simulink model "CryoDetHcd"  (R2016b)
settings: Solver=ode45  StartTime=0.0  StopTime=1e-3  RelTol=1e-3
PreLoadFcn:
  | setup_hcd
values from neighbouring files (symbols this model uses):
  A = sqrt(0.5*erfc(x))    [setup_hcd.m]
  etaRomData = zeros(1,128)    [setup_hcd.m]
  Fadc = 614e6    (= 614000000)    [setup_hcd.m]
  freqRomData = zeros(1,128)    [setup_hcd.m]
  freqRomData1 = zeros(1,128)    [setup_hcd.m]
  freqRomData2 = zeros(1,128)    [setup_hcd.m]
  freqRomData3 = zeros(1,128)    [setup_hcd.m]
undefined symbols (not defined in the file or in its folder): AXI4, B, C, D, j, Lite
libraries: xbsIndex_r4 x2151, CryoDetLibCMB x28, hdlsllib x8, dspsigops x2, simulink x1
(part 8 of 17)

== system CryoDetHcd/DspCore/DSP/channel_processor/channel_processor_x4/128_channel_processor1/DDS Mixer taylor series corrected ==
  rst : Inport
  In : Inport  Port=2
  freqBus : Inport  Port=3
  index : Inport  Port=4
  Bus Creator1 : BusCreator  Inputs=4
  Bus Creator2 : BusCreator  Inputs=5
  Bus Selector1 : BusSelector  OutputSignals=valid,Q,I,amp,ch
  Bus Selector2 : BusSelector  OutputSignals=valid
  Bus Selector : BusSelector  OutputSignals=freqWord,ch
  DDS 8ch taylor series corrected : Subsystem  AncestorBlock=CryoDetLibCMB/DDS 8ch taylor series corrected
  IQ_scale : CryoDetLibCMB/IQ_scale
  mixer : Subsystem
  tones : Outport
  downconvert : Outport  Port=2
  phase : Outport  Port=3
  wires:
  rst/1 -> DDS 8ch taylor series corrected/2(rst)
  Bus Selector/1 -> DDS 8ch taylor series corrected/3(freqWord)  "<freqWord>"
  Bus Selector1/5 -> IQ_scale/5  "<ch>"
  Bus Selector1/4 -> IQ_scale/4  "<amp>"
  DDS 8ch taylor series corrected/4(amp_o) -> Bus Creator2/4  "amp"
  DDS 8ch taylor series corrected/5(ch_o) -> Bus Creator2/5  "ch"
  In/1 -> Bus Selector2/1, mixer/2(In2)
  freqBus/1 -> Bus Selector/1
  Bus Selector2/1 -> DDS 8ch taylor series corrected/1(valid)  "<valid>"
  index/1 -> DDS 8ch taylor series corrected/4(index)
  IQ_scale/1 -> Bus Creator1/1  "valid"
  IQ_scale/2 -> Bus Creator1/2  "Q"
  IQ_scale/3 -> Bus Creator1/3  "I"
  IQ_scale/4 -> Bus Creator1/4  "ch"
  Bus Creator1/1 -> tones/1
  DDS 8ch taylor series corrected/3(I) -> Bus Creator2/3  "I"
  DDS 8ch taylor series corrected/1(valid_o) -> Bus Creator2/1  "valid"
  DDS 8ch taylor series corrected/2(Q) -> Bus Creator2/2  "Q"
  Bus Creator2/1 -> mixer/1(In1), Bus Selector1/1
  Bus Selector1/3 -> IQ_scale/3  "<I>"
  Bus Selector1/2 -> IQ_scale/2  "<Q>"
  Bus Selector1/1 -> IQ_scale/1  "<valid>"
  Bus Selector/2 -> DDS 8ch taylor series corrected/5(ch)  "<ch>"
  mixer/1(downmix) -> downconvert/1  "valid"
  mixer/2(phaseBus_o) -> phase/1
  DDS 8ch taylor series corrected/6(phaseBus) -> mixer/3(phaseBus)

== system CryoDetHcd/DspCore/DSP/channel_processor/channel_processor_x4/128_channel_processor1/IQ_status_sel ==
  sel : Inport
  Q : Inport  Port=2
  I : Inport  Port=3
  ch : Inport  Port=4
  BitBasher : xbsIndex_r4/BitBasher  bitexpr=out = {I,Q}  display_expr=off  sr_1=out  arith_type1=Unsigned  bin_pt1=0  sr_2=2  arith_type2=Unsigned  bin_pt2=0  sr_3=3  arith_type3=Unsigned  bin_pt3=0  sr_4=4  arith_type4=Unsigned  bin_pt4=0  dbl_ovrd=off  block_type=bitbasher
  Convert : xbsIndex_r4/Convert  gui_display_data_type=Fixed-point  arith_type="Signed  (2's comp)"  n_bits=16  bin_pt=15  float_type=Single  exp_bits=8  fraction_bits=24  quantization=Truncate  overflow=Wrap  en=off  latency=1  pipeline=off  dbl_ovrd=off  block_type=convert
  Convert1 : xbsIndex_r4/Convert  gui_display_data_type=Fixed-point  arith_type="Signed  (2's comp)"  n_bits=16  bin_pt=15  float_type=Single  exp_bits=8  fraction_bits=24  quantization=Truncate  overflow=Wrap  en=off  latency=1  pipeline=off  dbl_ovrd=off  block_type=convert
  Register1 : xbsIndex_r4/Register  init=0  rst=off  en=on  dbl_ovrd=off  block_type=register
  Relational : xbsIndex_r4/Relational  mode=a=b  op_type=Bool  en=off  latency=1  dbl_ovrd=off  block_type=relational
  IQ_status_r : Outport
  wires:
  sel/1 -> Relational/1
  Convert/1 -> BitBasher/1
  ch/1 -> Relational/2
  Q/1 -> Convert/1
  I/1 -> Convert1/1
  BitBasher/1 -> Register1/1
  Register1/1 -> IQ_status_r/1
  Convert1/1 -> BitBasher/2
  Relational/1 -> Register1/2

== system CryoDetHcd/DspCore/DSP/channel_processor/channel_processor_x4/128_channel_processor1/Variant Subsystem ==
  note: 1) Add Subsystem or Model blocks as valid variant choices.
      | 2) You cannot connect blocks at this level. At simulation, connectivity is automatically
      | determined, based on the active variant and port name matching.
  valid : Inport
  feedbackPolarity : Inport  Port=2
  feedbackGain : Inport  Port=3
  feedbackLimitHi : Inport  Port=4
  feedbackLimitLo : Inport  Port=5
  freqError : Inport  Port=6
  freqWord : Inport  Port=7
  ch : Inport  Port=8
  reset : Inport  Port=9
  LMS : Subsystem  AncestorBlock=CryoDetLibCMB/Loop Filter1  VariantControl=Variant
  Loop Filter1 : CryoDetLibCMB/Loop Filter1  VariantControl=Variant1
      link override Delay: rst=off  infoeditControl=Selection of Reset will increase slice count due to use of real FFs and instead of SRLs  en=off  latency=1  reg_retiming=off  dbl_ovrd=off
      link override Delay: infoedit=Hardware notes: A delay line is a chain, each link of which is an SRL16 followed by a flip-flop.
  valid_o : Outport
  freqWordOut : Outport  Port=2
  ch_o : Outport  Port=3

== system CryoDetHcd/DspCore/DSP/channel_processor/channel_processor_x4/128_channel_processor2/DDS Mixer taylor series corrected ==
  rst : Inport
  In : Inport  Port=2
  freqBus : Inport  Port=3
  index : Inport  Port=4
  Bus Creator1 : BusCreator  Inputs=4
  Bus Creator2 : BusCreator  Inputs=5
  Bus Selector1 : BusSelector  OutputSignals=valid,Q,I,amp,ch
  Bus Selector2 : BusSelector  OutputSignals=valid
  Bus Selector : BusSelector  OutputSignals=freqWord,ch
  DDS 8ch taylor series corrected : Subsystem  AncestorBlock=CryoDetLibCMB/DDS 8ch taylor series corrected
  IQ_scale : CryoDetLibCMB/IQ_scale
  mixer : Subsystem
  tones : Outport
  downconvert : Outport  Port=2
  phase : Outport  Port=3
  wires:
  DDS 8ch taylor series corrected/6(phaseBus) -> mixer/3(phaseBus)
  mixer/2(phaseBus_o) -> phase/1
  mixer/1(downmix) -> downconvert/1  "valid"
  Bus Selector/2 -> DDS 8ch taylor series corrected/5(ch)  "<ch>"
  Bus Selector1/1 -> IQ_scale/1  "<valid>"
  Bus Selector1/2 -> IQ_scale/2  "<Q>"
  Bus Selector1/3 -> IQ_scale/3  "<I>"
  Bus Creator2/1 -> Bus Selector1/1, mixer/1(In1)
  DDS 8ch taylor series corrected/2(Q) -> Bus Creator2/2  "Q"
  DDS 8ch taylor series corrected/1(valid_o) -> Bus Creator2/1  "valid"
  DDS 8ch taylor series corrected/3(I) -> Bus Creator2/3  "I"
  Bus Creator1/1 -> tones/1
  IQ_scale/4 -> Bus Creator1/4  "ch"
  IQ_scale/3 -> Bus Creator1/3  "I"
  IQ_scale/2 -> Bus Creator1/2  "Q"
  IQ_scale/1 -> Bus Creator1/1  "valid"
  index/1 -> DDS 8ch taylor series corrected/4(index)
  Bus Selector2/1 -> DDS 8ch taylor series corrected/1(valid)  "<valid>"
  freqBus/1 -> Bus Selector/1
  In/1 -> mixer/2(In2), Bus Selector2/1
  DDS 8ch taylor series corrected/5(ch_o) -> Bus Creator2/5  "ch"
  DDS 8ch taylor series corrected/4(amp_o) -> Bus Creator2/4  "amp"
  Bus Selector1/4 -> IQ_scale/4  "<amp>"
  Bus Selector1/5 -> IQ_scale/5  "<ch>"
  Bus Selector/1 -> DDS 8ch taylor series corrected/3(freqWord)  "<freqWord>"
  rst/1 -> DDS 8ch taylor series corrected/2(rst)

== system CryoDetHcd/DspCore/DSP/channel_processor/channel_processor_x4/128_channel_processor2/IQ_status_sel ==
  sel : Inport
  Q : Inport  Port=2
  I : Inport  Port=3
  ch : Inport  Port=4
  BitBasher : xbsIndex_r4/BitBasher  bitexpr=out = {I,Q}  display_expr=off  sr_1=out  arith_type1=Unsigned  bin_pt1=0  sr_2=2  arith_type2=Unsigned  bin_pt2=0  sr_3=3  arith_type3=Unsigned  bin_pt3=0  sr_4=4  arith_type4=Unsigned  bin_pt4=0  dbl_ovrd=off  block_type=bitbasher
  Convert : xbsIndex_r4/Convert  gui_display_data_type=Fixed-point  arith_type="Signed  (2's comp)"  n_bits=16  bin_pt=15  float_type=Single  exp_bits=8  fraction_bits=24  quantization=Truncate  overflow=Wrap  en=off  latency=1  pipeline=off  dbl_ovrd=off  block_type=convert
  Convert1 : xbsIndex_r4/Convert  gui_display_data_type=Fixed-point  arith_type="Signed  (2's comp)"  n_bits=16  bin_pt=15  float_type=Single  exp_bits=8  fraction_bits=24  quantization=Truncate  overflow=Wrap  en=off  latency=1  pipeline=off  dbl_ovrd=off  block_type=convert
  Register1 : xbsIndex_r4/Register  init=0  rst=off  en=on  dbl_ovrd=off  block_type=register
  Relational : xbsIndex_r4/Relational  mode=a=b  op_type=Bool  en=off  latency=1  dbl_ovrd=off  block_type=relational
  IQ_status_r : Outport
  wires:
  Relational/1 -> Register1/2
  Convert1/1 -> BitBasher/2
  Register1/1 -> IQ_status_r/1
  BitBasher/1 -> Register1/1
  I/1 -> Convert1/1
  Q/1 -> Convert/1
  ch/1 -> Relational/2
  Convert/1 -> BitBasher/1
  sel/1 -> Relational/1

== system CryoDetHcd/DspCore/DSP/channel_processor/channel_processor_x4/128_channel_processor2/Variant Subsystem ==
  note: 1) Add Subsystem or Model blocks as valid variant choices.
      | 2) You cannot connect blocks at this level. At simulation, connectivity is automatically
      | determined, based on the active variant and port name matching.
  valid : Inport
  feedbackPolarity : Inport  Port=2
  feedbackGain : Inport  Port=3
  feedbackLimitHi : Inport  Port=4
  feedbackLimitLo : Inport  Port=5
  freqError : Inport  Port=6
  freqWord : Inport  Port=7
  ch : Inport  Port=8
  reset : Inport  Port=9
  LMS : Subsystem  AncestorBlock=CryoDetLibCMB/Loop Filter1  VariantControl=Variant
  Loop Filter1 : CryoDetLibCMB/Loop Filter1  VariantControl=Variant1
      link override Delay: rst=off  infoeditControl=Selection of Reset will increase slice count due to use of real FFs and instead of SRLs  en=off  latency=1  reg_retiming=off  dbl_ovrd=off
      link override Delay: infoedit=Hardware notes: A delay line is a chain, each link of which is an SRL16 followed by a flip-flop.
  valid_o : Outport
  freqWordOut : Outport  Port=2
  ch_o : Outport  Port=3

== system CryoDetHcd/DspCore/DSP/channel_processor/channel_processor_x4/128_channel_processor3/DDS Mixer taylor series corrected ==
  rst : Inport
  In : Inport  Port=2
  freqBus : Inport  Port=3
  index : Inport  Port=4
  Bus Creator1 : BusCreator  Inputs=4
  Bus Creator2 : BusCreator  Inputs=5
  Bus Selector1 : BusSelector  OutputSignals=valid,Q,I,amp,ch
  Bus Selector2 : BusSelector  OutputSignals=valid
  Bus Selector : BusSelector  OutputSignals=freqWord,ch
  DDS 8ch taylor series corrected : Subsystem  AncestorBlock=CryoDetLibCMB/DDS 8ch taylor series corrected
  IQ_scale : CryoDetLibCMB/IQ_scale
  mixer : Subsystem
  tones : Outport
  downconvert : Outport  Port=2
  phase : Outport  Port=3
  wires:
  rst/1 -> DDS 8ch taylor series corrected/2(rst)
  Bus Selector/1 -> DDS 8ch taylor series corrected/3(freqWord)  "<freqWord>"
  Bus Selector1/5 -> IQ_scale/5  "<ch>"
  Bus Selector1/4 -> IQ_scale/4  "<amp>"
  DDS 8ch taylor series corrected/4(amp_o) -> Bus Creator2/4  "amp"
  DDS 8ch taylor series corrected/5(ch_o) -> Bus Creator2/5  "ch"
  In/1 -> Bus Selector2/1, mixer/2(In2)
  freqBus/1 -> Bus Selector/1
  Bus Selector2/1 -> DDS 8ch taylor series corrected/1(valid)  "<valid>"
  index/1 -> DDS 8ch taylor series corrected/4(index)
  IQ_scale/1 -> Bus Creator1/1  "valid"
  IQ_scale/2 -> Bus Creator1/2  "Q"
  IQ_scale/3 -> Bus Creator1/3  "I"
  IQ_scale/4 -> Bus Creator1/4  "ch"
  Bus Creator1/1 -> tones/1
  DDS 8ch taylor series corrected/3(I) -> Bus Creator2/3  "I"
  DDS 8ch taylor series corrected/1(valid_o) -> Bus Creator2/1  "valid"
  DDS 8ch taylor series corrected/2(Q) -> Bus Creator2/2  "Q"
  Bus Creator2/1 -> mixer/1(In1), Bus Selector1/1
  Bus Selector1/3 -> IQ_scale/3  "<I>"
  Bus Selector1/2 -> IQ_scale/2  "<Q>"
  Bus Selector1/1 -> IQ_scale/1  "<valid>"
  Bus Selector/2 -> DDS 8ch taylor series corrected/5(ch)  "<ch>"
  mixer/1(downmix) -> downconvert/1  "valid"
  mixer/2(phaseBus_o) -> phase/1
  DDS 8ch taylor series corrected/6(phaseBus) -> mixer/3(phaseBus)

== system CryoDetHcd/DspCore/DSP/channel_processor/channel_processor_x4/128_channel_processor3/IQ_status_sel ==
  sel : Inport
  Q : Inport  Port=2
  I : Inport  Port=3
  ch : Inport  Port=4
  BitBasher : xbsIndex_r4/BitBasher  bitexpr=out = {I,Q}  display_expr=off  sr_1=out  arith_type1=Unsigned  bin_pt1=0  sr_2=2  arith_type2=Unsigned  bin_pt2=0  sr_3=3  arith_type3=Unsigned  bin_pt3=0  sr_4=4  arith_type4=Unsigned  bin_pt4=0  dbl_ovrd=off  block_type=bitbasher
  Convert : xbsIndex_r4/Convert  gui_display_data_type=Fixed-point  arith_type="Signed  (2's comp)"  n_bits=16  bin_pt=15  float_type=Single  exp_bits=8  fraction_bits=24  quantization=Truncate  overflow=Wrap  en=off  latency=1  pipeline=off  dbl_ovrd=off  block_type=convert
  Convert1 : xbsIndex_r4/Convert  gui_display_data_type=Fixed-point  arith_type="Signed  (2's comp)"  n_bits=16  bin_pt=15  float_type=Single  exp_bits=8  fraction_bits=24  quantization=Truncate  overflow=Wrap  en=off  latency=1  pipeline=off  dbl_ovrd=off  block_type=convert
  Register1 : xbsIndex_r4/Register  init=0  rst=off  en=on  dbl_ovrd=off  block_type=register
  Relational : xbsIndex_r4/Relational  mode=a=b  op_type=Bool  en=off  latency=1  dbl_ovrd=off  block_type=relational
  IQ_status_r : Outport
  wires:
  sel/1 -> Relational/1
  Convert/1 -> BitBasher/1
  ch/1 -> Relational/2
  Q/1 -> Convert/1
  I/1 -> Convert1/1
  BitBasher/1 -> Register1/1
  Register1/1 -> IQ_status_r/1
  Convert1/1 -> BitBasher/2
  Relational/1 -> Register1/2

== system CryoDetHcd/DspCore/DSP/channel_processor/channel_processor_x4/128_channel_processor3/Variant Subsystem ==
  note: 1) Add Subsystem or Model blocks as valid variant choices.
      | 2) You cannot connect blocks at this level. At simulation, connectivity is automatically
      | determined, based on the active variant and port name matching.
  valid : Inport
  feedbackPolarity : Inport  Port=2
  feedbackGain : Inport  Port=3
  feedbackLimitHi : Inport  Port=4
  feedbackLimitLo : Inport  Port=5
  freqError : Inport  Port=6
  freqWord : Inport  Port=7
  ch : Inport  Port=8
  reset : Inport  Port=9
  LMS : Subsystem  AncestorBlock=CryoDetLibCMB/Loop Filter1  VariantControl=Variant
  Loop Filter1 : CryoDetLibCMB/Loop Filter1  VariantControl=Variant1
      link override Delay: rst=off  infoeditControl=Selection of Reset will increase slice count due to use of real FFs and instead of SRLs  en=off  latency=1  reg_retiming=off  dbl_ovrd=off
      link override Delay: infoedit=Hardware notes: A delay line is a chain, each link of which is an SRL16 followed by a flip-flop.
  valid_o : Outport
  freqWordOut : Outport  Port=2
  ch_o : Outport  Port=3

== system CryoDetHcd/DspCore/DSP/channel_processor/channel_processor_x4/128_channel_processor4/DDS Mixer taylor series corrected ==
  rst : Inport
  In : Inport  Port=2
  freqBus : Inport  Port=3
  index : Inport  Port=4
  Bus Creator1 : BusCreator  Inputs=4
  Bus Creator2 : BusCreator  Inputs=5
  Bus Selector1 : BusSelector  OutputSignals=valid,Q,I,amp,ch
  Bus Selector2 : BusSelector  OutputSignals=valid
  Bus Selector : BusSelector  OutputSignals=freqWord,ch
  DDS 8ch taylor series corrected : Subsystem  AncestorBlock=CryoDetLibCMB/DDS 8ch taylor series corrected
  IQ_scale : CryoDetLibCMB/IQ_scale
  mixer : Subsystem
  tones : Outport
  downconvert : Outport  Port=2
  phase : Outport  Port=3
  wires:
  DDS 8ch taylor series corrected/6(phaseBus) -> mixer/3(phaseBus)
  mixer/2(phaseBus_o) -> phase/1
  mixer/1(downmix) -> downconvert/1  "valid"
  Bus Selector/2 -> DDS 8ch taylor series corrected/5(ch)  "<ch>"
  Bus Selector1/1 -> IQ_scale/1  "<valid>"
  Bus Selector1/2 -> IQ_scale/2  "<Q>"
  Bus Selector1/3 -> IQ_scale/3  "<I>"
  Bus Creator2/1 -> Bus Selector1/1, mixer/1(In1)
  DDS 8ch taylor series corrected/2(Q) -> Bus Creator2/2  "Q"
  DDS 8ch taylor series corrected/1(valid_o) -> Bus Creator2/1  "valid"
  DDS 8ch taylor series corrected/3(I) -> Bus Creator2/3  "I"
  Bus Creator1/1 -> tones/1
  IQ_scale/4 -> Bus Creator1/4  "ch"
  IQ_scale/3 -> Bus Creator1/3  "I"
  IQ_scale/2 -> Bus Creator1/2  "Q"
  IQ_scale/1 -> Bus Creator1/1  "valid"
  index/1 -> DDS 8ch taylor series corrected/4(index)
  Bus Selector2/1 -> DDS 8ch taylor series corrected/1(valid)  "<valid>"
  freqBus/1 -> Bus Selector/1
  In/1 -> mixer/2(In2), Bus Selector2/1
  DDS 8ch taylor series corrected/5(ch_o) -> Bus Creator2/5  "ch"
  DDS 8ch taylor series corrected/4(amp_o) -> Bus Creator2/4  "amp"
  Bus Selector1/4 -> IQ_scale/4  "<amp>"
  Bus Selector1/5 -> IQ_scale/5  "<ch>"
  Bus Selector/1 -> DDS 8ch taylor series corrected/3(freqWord)  "<freqWord>"
  rst/1 -> DDS 8ch taylor series corrected/2(rst)

== system CryoDetHcd/DspCore/DSP/channel_processor/channel_processor_x4/128_channel_processor4/IQ_status_sel ==
  sel : Inport
  Q : Inport  Port=2
  I : Inport  Port=3
  ch : Inport  Port=4
  BitBasher : xbsIndex_r4/BitBasher  bitexpr=out = {I,Q}  display_expr=off  sr_1=out  arith_type1=Unsigned  bin_pt1=0  sr_2=2  arith_type2=Unsigned  bin_pt2=0  sr_3=3  arith_type3=Unsigned  bin_pt3=0  sr_4=4  arith_type4=Unsigned  bin_pt4=0  dbl_ovrd=off  block_type=bitbasher
  Convert : xbsIndex_r4/Convert  gui_display_data_type=Fixed-point  arith_type="Signed  (2's comp)"  n_bits=16  bin_pt=15  float_type=Single  exp_bits=8  fraction_bits=24  quantization=Truncate  overflow=Wrap  en=off  latency=1  pipeline=off  dbl_ovrd=off  block_type=convert
  Convert1 : xbsIndex_r4/Convert  gui_display_data_type=Fixed-point  arith_type="Signed  (2's comp)"  n_bits=16  bin_pt=15  float_type=Single  exp_bits=8  fraction_bits=24  quantization=Truncate  overflow=Wrap  en=off  latency=1  pipeline=off  dbl_ovrd=off  block_type=convert
  Register1 : xbsIndex_r4/Register  init=0  rst=off  en=on  dbl_ovrd=off  block_type=register
  Relational : xbsIndex_r4/Relational  mode=a=b  op_type=Bool  en=off  latency=1  dbl_ovrd=off  block_type=relational
  IQ_status_r : Outport
  wires:
  Relational/1 -> Register1/2
  Convert1/1 -> BitBasher/2
  Register1/1 -> IQ_status_r/1
  BitBasher/1 -> Register1/1
  I/1 -> Convert1/1
  Q/1 -> Convert/1
  ch/1 -> Relational/2
  Convert/1 -> BitBasher/1
  sel/1 -> Relational/1

== system CryoDetHcd/DspCore/DSP/channel_processor/channel_processor_x4/128_channel_processor4/Variant Subsystem ==
  note: 1) Add Subsystem or Model blocks as valid variant choices.
      | 2) You cannot connect blocks at this level. At simulation, connectivity is automatically
      | determined, based on the active variant and port name matching.
  valid : Inport
  feedbackPolarity : Inport  Port=2
  feedbackGain : Inport  Port=3
  feedbackLimitHi : Inport  Port=4
  feedbackLimitLo : Inport  Port=5
  freqError : Inport  Port=6
  freqWord : Inport  Port=7
  ch : Inport  Port=8
  reset : Inport  Port=9
  LMS : Subsystem  AncestorBlock=CryoDetLibCMB/Loop Filter1  VariantControl=Variant
  Loop Filter1 : CryoDetLibCMB/Loop Filter1  VariantControl=Variant1
      link override Delay: rst=off  infoeditControl=Selection of Reset will increase slice count due to use of real FFs and instead of SRLs  en=off  latency=1  reg_retiming=off  dbl_ovrd=off
      link override Delay: infoedit=Hardware notes: A delay line is a chain, each link of which is an SRL16 followed by a flip-flop.
  valid_o : Outport
  freqWordOut : Outport  Port=2
  ch_o : Outport  Port=3

== system CryoDetHcd/DspCore/DSP/channel_processor/channel_processor_x4/dF_debug/alpha_filter ==
  In1 : Inport
  alpha : Inport  Port=2
  ch : Inport  Port=3
  (D-A)*B + C : xbsIndex_r4/DSP48 Macro 3.0   dsptype=Target XtremeDSP Slice: DSP48E2  instruction_list=(D-A)*B+C  AvailableInstructions=|  show_filtered=on  pipeline_options=Expert  dspimage=?  tier_1=off  tier_2=off  tier_3=off  tier_4=off  tier_5=off  tier_6=off  dreg_1=off  dreg_2=off  dreg_3=on  areg_1=off  areg_2=off  areg_3=on  areg_4=on  breg_1=off  breg_2=off  breg_3=on  breg_4=on  mreg_5=on  concatreg_3=off  concatreg_4=off  concatreg_5=off  creg_1=off  creg_2=off  creg_3=on  creg_4=on  creg_5=on  preg_6=on  cinreg_1=off  cinreg_2=off  cinreg_3=off  cinreg_4=off  cinreg_5=off  opreg_1=off  opreg_2=off  opreg_3=off  opreg_4=off  opreg_5=off  output_properties=Full_Precision  p_width=48  p_binarywidth=0  has_acout=off  has_bcout=off  has_pcout=off  has_carryout=off  has_carrycascout=off  has_ce=off  has_d_ce=off  has_a_ce=off  has_b_ce=off  has_concat_ce=off  has_c_ce=off  has_m_ce=off  has_p_ce=off  has_sel_ce=off  has_sclr=off  has_d_sclr=off  has_a_sclr=off  has_b_sclr=off  has_concat_sclr=off  has_c_sclr=off  has_m_sclr=off  has_p_sclr=off  has_sel_sclr=off  use_dsp48=on  simulation_type=fast_sim  simulation_model=sysgen:xbip_dsp48_macro_v3_0  gui_behaviour=Sysgen  instruction1='#'  ip_name=DSP48 Macro  ip_version=3.0  dsptool_ready=true  ipcore_usecache=true  ipcore_useipmodelcache=true  wrapper_available=true  port_translation_map={ 'ce' => 'en', 'sclr' => 'rst'}  ipcore_latency_function='has_combinational'  structural_sim=false  ipcore_verbose=false  ipcore_port_config={ 'carryin' => { 'arith' => 'ufix', 'binpt' => 0.00000000000, 'width' => 1.00000000000}, 'carrycascin' => { 'arith' => 'ufix', 'binpt' => 0.00000000000, 'width' => 1.00000000000}, 'carrycascout' => { 'arith' => 'ufix', 'binpt' => 0.00000000000, 'width' => 1.00000000000}, 'carryout' => { 'arith' => 'ufix', 'binpt' => 0.00000000000, 'width' => 1.00000000000}}  ipcore_xco_need_fpga_part=true  block_type=xbip_dsp48_macro_v3_0
      | (D-A)*B+C
      | (D-A)*B+C+C
      | (D-A)*B+C+C+CARRYIN
      | (D-A)*B+C+CARRYIN
      | (D-A)*B+C+P
      | (D-A)*B+C+P+CARRYIN
      | (D-A)*B+C+P>>17
      | (D-A)*B+C+P>>17+CARRYIN
      | (D-A)*B+C+PCIN
      | (D-A)*B+C+PCIN+CARRYIN
      | (D-A)*B+C+PCIN>>17
      | (D-A)*B+C+PCIN>>17+CARRYIN
      | (D-A)*B+C-C
      | (D-A)*B+C-P
      | (D-A)*B+C-P>>17
      | (D-A)*B+C-PCIN
      | (D-A)*B+C-PCIN>>17
      | (D-A)*B+CARRYIN
      | -((D-A)*B+C)
      | -((D-A)*B+C+CARRYIN)
      | -((D-A)*B+CARRYIN)
      | -(C+(D-A)*B+CARRYIN)
      | -(P+(D-A)*B+CARRYIN)
      | -C+(D-A)*B+C
      | -P+(D-A)*B+C
      | -P>>17+(D-A)*B+C
      | -PCIN+(D-A)*B+C
      | -PCIN>>17+(D-A)*B+C
      | C+(D-A)*B+C
      | C+(D-A)*B+C+CARRYIN
      | C+(D-A)*B+CARRYIN
      | C+C+(D-A)*B+CARRYIN
      | C+P+(D-A)*B+CARRYIN
      | C+P>>17+(D-A)*B+CARRYIN
      | C+PCIN+(D-A)*B+CARRYIN
      | C+PCIN>>17+(D-A)*B+CARRYIN
      | C-((D-A)*B+C)
      | C-((D-A)*B+C+CARRYIN)
      | C-((D-A)*B+CARRYIN)
      | C-(C+(D-A)*B+CARRYIN)
      | C-(P+(D-A)*B+CARRYIN)
      | P+(D-A)*B+C
      | P+(D-A)*B+C+CARRYIN
      | P+(D-A)*B+CARRYIN
      | P+C+(D-A)*B+CARRYIN
      | P+P+(D-A)*B+CARRYIN
      | P+P>>17+(D-A)*B+CARRYIN
      | P+PCIN+(D-A)*B+CARRYIN
      | P+PCIN>>17+(D-A)*B+CARRYIN
      | P-((D-A)*B+C)
      | P-((D-A)*B+C+CARRYIN)
      | P-((D-A)*B+CARRYIN)
      | P-(C+(D-A)*B+CARRYIN)
      | P-(P+(D-A)*B+CARRYIN)
      | P>>17+(D-A)*B+C
      | P>>17+(D-A)*B+C+CARRYIN
      | P>>17+(D-A)*B+CARRYIN
      | P>>17+C+(D-A)*B+CARRYIN
      | P>>17+P+(D-A)*B+CARRYIN
      | P>>17-((D-A)*B+C)
      | P>>17-((D-A)*B+C+CARRYIN)
      | P>>17-((D-A)*B+CARRYIN)
      | P>>17-(C+(D-A)*B+CARRYIN)
      | P>>17-(P+(D-A)*B+CARRYIN)
      | PCIN+(D-A)*B+C
      | PCIN+(D-A)*B+C+CARRYIN
      | PCIN+(D-A)*B+CARRYIN
      | PCIN+C+(D-A)*B+CARRYIN
      | PCIN+P+(D-A)*B+CARRYIN
      | PCIN-((D-A)*B+C)
      | PCIN-((D-A)*B+C+CARRYIN)
      | PCIN-((D-A)*B+CARRYIN)
      | PCIN-(C+(D-A)*B+CARRYIN)
      | PCIN-(P+(D-A)*B+CARRYIN)
      | PCIN>>17+(D-A)*B+C
      | PCIN>>17+(D-A)*B+C+CARRYIN
      | PCIN>>17+(D-A)*B+CARRYIN
      | PCIN>>17+C+(D-A)*B+CARRYIN
      | PCIN>>17+P+(D-A)*B+CARRYIN
      | PCIN>>17-((D-A)*B+C)
      | PCIN>>17-((D-A)*B+C+CARRYIN)
      | PCIN>>17-((D-A)*B+CARRYIN)
      | PCIN>>17-(C+(D-A)*B+CARRYIN)
      | PCIN>>17-(P+(D-A)*B+CARRYIN)
      | RNDMACC((D-A)*B+C+P)
      | RNDSIMPLE((D-A)*B+C)
      | RNDSIMPLE((D-A)*B+C+CARRYIN)
      | RNDSIMPLE((D-A)*B+CARRYIN)
      | RNDSIMPLE(C+(D-A)*B+CARRYIN)
      | RNDSIMPLE(P+(D-A)*B+CARRYIN)
      | RNDSIMPLE(P>>17+(D-A)*B+CARRYIN)
      | RNDSIMPLE(PCIN+(D-A)*B+CARRYIN)
      | RNDSIMPLE(PCIN>>17+(D-A)*B+CARRYIN)
      settings: infoedit=<html>Valid operands: CONCAT, P, C, PCIN, P>>17, PCIN>>17, CARRYIN, CARRYCASCIN, ACIN, A, BCIN,B<br><br>Valid operators: +, -, *, ()<br><br>Valid functions: RNDSIMPLE, RNDSYM<br><br>Instructions are case insensitive and tolerate spaces.</html>
  Convert : xbsIndex_r4/Convert  gui_display_data_type=Fixed-point  arith_type=Unsigned  n_bits=24  bin_pt=0  float_type=Single  exp_bits=8  fraction_bits=24  quantization=Truncate  overflow=Wrap  en=off  latency=0  pipeline=off  dbl_ovrd=off  block_type=convert
  Convert1 : xbsIndex_r4/Convert  gui_display_data_type=Fixed-point  arith_type="Signed  (2's comp)"  n_bits=25  bin_pt=0  float_type=Single  exp_bits=8  fraction_bits=24  quantization=Truncate  overflow=Wrap  en=off  latency=0  pipeline=off  dbl_ovrd=off  block_type=convert
  Convert2 : xbsIndex_r4/Convert  gui_display_data_type=Fixed-point  arith_type="Signed  (2's comp)"  n_bits=18  bin_pt=15  float_type=Single  exp_bits=8  fraction_bits=24  quantization=Truncate  overflow=Wrap  en=off  latency=0  pipeline=off  dbl_ovrd=off  block_type=convert
  Convert3 : xbsIndex_r4/Convert  gui_display_data_type=Fixed-point  arith_type="Signed  (2's comp)"  n_bits=25  bin_pt=0  float_type=Single  exp_bits=8  fraction_bits=24  quantization=Truncate  overflow=Wrap  en=off  latency=0  pipeline=off  dbl_ovrd=off  block_type=convert
  Delay : xbsIndex_r4/Delay  rst=off  infoeditControl=Selection of Reset will increase slice count due to use of real FFs and instead of SRLs  en=off  latency=4  reg_retiming=off  dbl_ovrd=off  block_type=delay
  Delay1 : xbsIndex_r4/Delay  rst=off  infoeditControl=Selection of Reset will increase slice count due to use of real FFs and instead of SRLs  en=off  latency=4  reg_retiming=off  dbl_ovrd=off  block_type=delay
  Register : xbsIndex_r4/Register  init=0  rst=off  en=off  dbl_ovrd=off  block_type=register
  Out1 : Outport
  ch_o : Outport  Port=2
  wires:
  Register/1 -> Convert3/1
  In1/1 -> Register/1
  Delay/1 -> Convert1/1, (D-A)*B + C/4
  (D-A)*B + C/1 -> Convert/1, Delay/1
  Convert1/1 -> (D-A)*B + C/2
  Convert/1 -> Out1/1
  Convert2/1 -> (D-A)*B + C/3
  Convert3/1 -> (D-A)*B + C/1
  ch/1 -> Delay1/1
  Delay1/1 -> ch_o/1
  alpha/1 -> Convert2/1

== system CryoDetHcd/DspCore/DSP/channel_processor/channel_processor_x4/dF_debug/alpha_filter1 ==
  In1 : Inport
  alpha : Inport  Port=2
  ch : Inport  Port=3
  (D-A)*B + C : xbsIndex_r4/DSP48 Macro 3.0   dsptype=Target XtremeDSP Slice: DSP48E2  instruction_list=(D-A)*B+C  AvailableInstructions=|  show_filtered=on  pipeline_options=Expert  dspimage=?  tier_1=off  tier_2=off  tier_3=off  tier_4=off  tier_5=off  tier_6=off  dreg_1=off  dreg_2=off  dreg_3=on  areg_1=off  areg_2=off  areg_3=on  areg_4=on  breg_1=off  breg_2=off  breg_3=on  breg_4=on  mreg_5=on  concatreg_3=off  concatreg_4=off  concatreg_5=off  creg_1=off  creg_2=off  creg_3=on  creg_4=on  creg_5=on  preg_6=on  cinreg_1=off  cinreg_2=off  cinreg_3=off  cinreg_4=off  cinreg_5=off  opreg_1=off  opreg_2=off  opreg_3=off  opreg_4=off  opreg_5=off  output_properties=Full_Precision  p_width=48  p_binarywidth=0  has_acout=off  has_bcout=off  has_pcout=off  has_carryout=off  has_carrycascout=off  has_ce=off  has_d_ce=off  has_a_ce=off  has_b_ce=off  has_concat_ce=off  has_c_ce=off  has_m_ce=off  has_p_ce=off  has_sel_ce=off  has_sclr=off  has_d_sclr=off  has_a_sclr=off  has_b_sclr=off  has_concat_sclr=off  has_c_sclr=off  has_m_sclr=off  has_p_sclr=off  has_sel_sclr=off  use_dsp48=on  simulation_type=fast_sim  simulation_model=sysgen:xbip_dsp48_macro_v3_0  gui_behaviour=Sysgen  instruction1='#'  ip_name=DSP48 Macro  ip_version=3.0  dsptool_ready=true  ipcore_usecache=true  ipcore_useipmodelcache=true  wrapper_available=true  port_translation_map={ 'ce' => 'en', 'sclr' => 'rst'}  ipcore_latency_function='has_combinational'  structural_sim=false  ipcore_verbose=false  ipcore_port_config={ 'carryin' => { 'arith' => 'ufix', 'binpt' => 0.00000000000, 'width' => 1.00000000000}, 'carrycascin' => { 'arith' => 'ufix', 'binpt' => 0.00000000000, 'width' => 1.00000000000}, 'carrycascout' => { 'arith' => 'ufix', 'binpt' => 0.00000000000, 'width' => 1.00000000000}, 'carryout' => { 'arith' => 'ufix', 'binpt' => 0.00000000000, 'width' => 1.00000000000}}  ipcore_xco_need_fpga_part=true  block_type=xbip_dsp48_macro_v3_0
      | (D-A)*B+C
      | (D-A)*B+C+C
      | (D-A)*B+C+C+CARRYIN
      | (D-A)*B+C+CARRYIN
      | (D-A)*B+C+P
      | (D-A)*B+C+P+CARRYIN
      | (D-A)*B+C+P>>17
      | (D-A)*B+C+P>>17+CARRYIN
      | (D-A)*B+C+PCIN
      | (D-A)*B+C+PCIN+CARRYIN
      | (D-A)*B+C+PCIN>>17
      | (D-A)*B+C+PCIN>>17+CARRYIN
      | (D-A)*B+C-C
      | (D-A)*B+C-P
      | (D-A)*B+C-P>>17
      | (D-A)*B+C-PCIN
      | (D-A)*B+C-PCIN>>17
      | (D-A)*B+CARRYIN
      | -((D-A)*B+C)
      | -((D-A)*B+C+CARRYIN)
      | -((D-A)*B+CARRYIN)
      | -(C+(D-A)*B+CARRYIN)
      | -(P+(D-A)*B+CARRYIN)
      | -C+(D-A)*B+C
      | -P+(D-A)*B+C
      | -P>>17+(D-A)*B+C
      | -PCIN+(D-A)*B+C
      | -PCIN>>17+(D-A)*B+C
      | C+(D-A)*B+C
      | C+(D-A)*B+C+CARRYIN
      | C+(D-A)*B+CARRYIN
      | C+C+(D-A)*B+CARRYIN
      | C+P+(D-A)*B+CARRYIN
      | C+P>>17+(D-A)*B+CARRYIN
      | C+PCIN+(D-A)*B+CARRYIN
      | C+PCIN>>17+(D-A)*B+CARRYIN
      | C-((D-A)*B+C)
      | C-((D-A)*B+C+CARRYIN)
      | C-((D-A)*B+CARRYIN)
      | C-(C+(D-A)*B+CARRYIN)
      | C-(P+(D-A)*B+CARRYIN)
      | P+(D-A)*B+C
      | P+(D-A)*B+C+CARRYIN
      | P+(D-A)*B+CARRYIN
      | P+C+(D-A)*B+CARRYIN
      | P+P+(D-A)*B+CARRYIN
      | P+P>>17+(D-A)*B+CARRYIN
      | P+PCIN+(D-A)*B+CARRYIN
      | P+PCIN>>17+(D-A)*B+CARRYIN
      | P-((D-A)*B+C)
      | P-((D-A)*B+C+CARRYIN)
      | P-((D-A)*B+CARRYIN)
      | P-(C+(D-A)*B+CARRYIN)
      | P-(P+(D-A)*B+CARRYIN)
      | P>>17+(D-A)*B+C
      | P>>17+(D-A)*B+C+CARRYIN
      | P>>17+(D-A)*B+CARRYIN
      | P>>17+C+(D-A)*B+CARRYIN
      | P>>17+P+(D-A)*B+CARRYIN
      | P>>17-((D-A)*B+C)
      | P>>17-((D-A)*B+C+CARRYIN)
      | P>>17-((D-A)*B+CARRYIN)
      | P>>17-(C+(D-A)*B+CARRYIN)
      | P>>17-(P+(D-A)*B+CARRYIN)
      | PCIN+(D-A)*B+C
      | PCIN+(D-A)*B+C+CARRYIN
      | PCIN+(D-A)*B+CARRYIN
      | PCIN+C+(D-A)*B+CARRYIN
      | PCIN+P+(D-A)*B+CARRYIN
      | PCIN-((D-A)*B+C)
      | PCIN-((D-A)*B+C+CARRYIN)
      | PCIN-((D-A)*B+CARRYIN)
      | PCIN-(C+(D-A)*B+CARRYIN)
      | PCIN-(P+(D-A)*B+CARRYIN)
      | PCIN>>17+(D-A)*B+C
      | PCIN>>17+(D-A)*B+C+CARRYIN
      | PCIN>>17+(D-A)*B+CARRYIN
      | PCIN>>17+C+(D-A)*B+CARRYIN
      | PCIN>>17+P+(D-A)*B+CARRYIN
      | PCIN>>17-((D-A)*B+C)
      | PCIN>>17-((D-A)*B+C+CARRYIN)
      | PCIN>>17-((D-A)*B+CARRYIN)
      | PCIN>>17-(C+(D-A)*B+CARRYIN)
      | PCIN>>17-(P+(D-A)*B+CARRYIN)
      | RNDMACC((D-A)*B+C+P)
      | RNDSIMPLE((D-A)*B+C)
      | RNDSIMPLE((D-A)*B+C+CARRYIN)
      | RNDSIMPLE((D-A)*B+CARRYIN)
      | RNDSIMPLE(C+(D-A)*B+CARRYIN)
      | RNDSIMPLE(P+(D-A)*B+CARRYIN)
      | RNDSIMPLE(P>>17+(D-A)*B+CARRYIN)
      | RNDSIMPLE(PCIN+(D-A)*B+CARRYIN)
      | RNDSIMPLE(PCIN>>17+(D-A)*B+CARRYIN)
      settings: infoedit=<html>Valid operands: CONCAT, P, C, PCIN, P>>17, PCIN>>17, CARRYIN, CARRYCASCIN, ACIN, A, BCIN,B<br><br>Valid operators: +, -, *, ()<br><br>Valid functions: RNDSIMPLE, RNDSYM<br><br>Instructions are case insensitive and tolerate spaces.</html>
  Convert : xbsIndex_r4/Convert  gui_display_data_type=Fixed-point  arith_type=Unsigned  n_bits=24  bin_pt=0  float_type=Single  exp_bits=8  fraction_bits=24  quantization=Truncate  overflow=Wrap  en=off  latency=0  pipeline=off  dbl_ovrd=off  block_type=convert
  Convert1 : xbsIndex_r4/Convert  gui_display_data_type=Fixed-point  arith_type="Signed  (2's comp)"  n_bits=25  bin_pt=0  float_type=Single  exp_bits=8  fraction_bits=24  quantization=Truncate  overflow=Wrap  en=off  latency=0  pipeline=off  dbl_ovrd=off  block_type=convert
  Convert2 : xbsIndex_r4/Convert  gui_display_data_type=Fixed-point  arith_type="Signed  (2's comp)"  n_bits=18  bin_pt=15  float_type=Single  exp_bits=8  fraction_bits=24  quantization=Truncate  overflow=Wrap  en=off  latency=0  pipeline=off  dbl_ovrd=off  block_type=convert
  Convert3 : xbsIndex_r4/Convert  gui_display_data_type=Fixed-point  arith_type="Signed  (2's comp)"  n_bits=25  bin_pt=0  float_type=Single  exp_bits=8  fraction_bits=24  quantization=Truncate  overflow=Wrap  en=off  latency=0  pipeline=off  dbl_ovrd=off  block_type=convert
  Delay : xbsIndex_r4/Delay  rst=off  infoeditControl=Selection of Reset will increase slice count due to use of real FFs and instead of SRLs  en=off  latency=4  reg_retiming=off  dbl_ovrd=off  block_type=delay
  Delay1 : xbsIndex_r4/Delay  rst=off  infoeditControl=Selection of Reset will increase slice count due to use of real FFs and instead of SRLs  en=off  latency=4  reg_retiming=off  dbl_ovrd=off  block_type=delay
  Register : xbsIndex_r4/Register  init=0  rst=off  en=off  dbl_ovrd=off  block_type=register
  Out1 : Outport
  ch_o : Outport  Port=2
  wires:
  alpha/1 -> Convert2/1
  Delay1/1 -> ch_o/1
  ch/1 -> Delay1/1
  Convert3/1 -> (D-A)*B + C/1
  Convert2/1 -> (D-A)*B + C/3
  Convert/1 -> Out1/1
  Convert1/1 -> (D-A)*B + C/2
  (D-A)*B + C/1 -> Delay/1, Convert/1
  Delay/1 -> (D-A)*B + C/4, Convert1/1
  In1/1 -> Register/1
  Register/1 -> Convert3/1

== system CryoDetHcd/DspCore/DSP/channel_processor/channel_processor_x4/dF_debug/alpha_filter2 ==
  In1 : Inport
  alpha : Inport  Port=2
  ch : Inport  Port=3
  (D-A)*B + C : xbsIndex_r4/DSP48 Macro 3.0   dsptype=Target XtremeDSP Slice: DSP48E2  instruction_list=(D-A)*B+C  AvailableInstructions=|  show_filtered=on  pipeline_options=Expert  dspimage=?  tier_1=off  tier_2=off  tier_3=off  tier_4=off  tier_5=off  tier_6=off  dreg_1=off  dreg_2=off  dreg_3=on  areg_1=off  areg_2=off  areg_3=on  areg_4=on  breg_1=off  breg_2=off  breg_3=on  breg_4=on  mreg_5=on  concatreg_3=off  concatreg_4=off  concatreg_5=off  creg_1=off  creg_2=off  creg_3=on  creg_4=on  creg_5=on  preg_6=on  cinreg_1=off  cinreg_2=off  cinreg_3=off  cinreg_4=off  cinreg_5=off  opreg_1=off  opreg_2=off  opreg_3=off  opreg_4=off  opreg_5=off  output_properties=Full_Precision  p_width=48  p_binarywidth=0  has_acout=off  has_bcout=off  has_pcout=off  has_carryout=off  has_carrycascout=off  has_ce=off  has_d_ce=off  has_a_ce=off  has_b_ce=off  has_concat_ce=off  has_c_ce=off  has_m_ce=off  has_p_ce=off  has_sel_ce=off  has_sclr=off  has_d_sclr=off  has_a_sclr=off  has_b_sclr=off  has_concat_sclr=off  has_c_sclr=off  has_m_sclr=off  has_p_sclr=off  has_sel_sclr=off  use_dsp48=on  simulation_type=fast_sim  simulation_model=sysgen:xbip_dsp48_macro_v3_0  gui_behaviour=Sysgen  instruction1='#'  ip_name=DSP48 Macro  ip_version=3.0  dsptool_ready=true  ipcore_usecache=true  ipcore_useipmodelcache=true  wrapper_available=true  port_translation_map={ 'ce' => 'en', 'sclr' => 'rst'}  ipcore_latency_function='has_combinational'  structural_sim=false  ipcore_verbose=false  ipcore_port_config={ 'carryin' => { 'arith' => 'ufix', 'binpt' => 0.00000000000, 'width' => 1.00000000000}, 'carrycascin' => { 'arith' => 'ufix', 'binpt' => 0.00000000000, 'width' => 1.00000000000}, 'carrycascout' => { 'arith' => 'ufix', 'binpt' => 0.00000000000, 'width' => 1.00000000000}, 'carryout' => { 'arith' => 'ufix', 'binpt' => 0.00000000000, 'width' => 1.00000000000}}  ipcore_xco_need_fpga_part=true  block_type=xbip_dsp48_macro_v3_0
      | (D-A)*B+C
      | (D-A)*B+C+C
      | (D-A)*B+C+C+CARRYIN
      | (D-A)*B+C+CARRYIN
      | (D-A)*B+C+P
      | (D-A)*B+C+P+CARRYIN
      | (D-A)*B+C+P>>17
      | (D-A)*B+C+P>>17+CARRYIN
      | (D-A)*B+C+PCIN
      | (D-A)*B+C+PCIN+CARRYIN
      | (D-A)*B+C+PCIN>>17
      | (D-A)*B+C+PCIN>>17+CARRYIN
      | (D-A)*B+C-C
      | (D-A)*B+C-P
      | (D-A)*B+C-P>>17
      | (D-A)*B+C-PCIN
      | (D-A)*B+C-PCIN>>17
      | (D-A)*B+CARRYIN
      | -((D-A)*B+C)
      | -((D-A)*B+C+CARRYIN)
      | -((D-A)*B+CARRYIN)
      | -(C+(D-A)*B+CARRYIN)
      | -(P+(D-A)*B+CARRYIN)
      | -C+(D-A)*B+C
      | -P+(D-A)*B+C
      | -P>>17+(D-A)*B+C
      | -PCIN+(D-A)*B+C
      | -PCIN>>17+(D-A)*B+C
      | C+(D-A)*B+C
      | C+(D-A)*B+C+CARRYIN
      | C+(D-A)*B+CARRYIN
      | C+C+(D-A)*B+CARRYIN
      | C+P+(D-A)*B+CARRYIN
      | C+P>>17+(D-A)*B+CARRYIN
      | C+PCIN+(D-A)*B+CARRYIN
      | C+PCIN>>17+(D-A)*B+CARRYIN
      | C-((D-A)*B+C)
      | C-((D-A)*B+C+CARRYIN)
      | C-((D-A)*B+CARRYIN)
      | C-(C+(D-A)*B+CARRYIN)
      | C-(P+(D-A)*B+CARRYIN)
      | P+(D-A)*B+C
      | P+(D-A)*B+C+CARRYIN
      | P+(D-A)*B+CARRYIN
      | P+C+(D-A)*B+CARRYIN
      | P+P+(D-A)*B+CARRYIN
      | P+P>>17+(D-A)*B+CARRYIN
      | P+PCIN+(D-A)*B+CARRYIN
      | P+PCIN>>17+(D-A)*B+CARRYIN
      | P-((D-A)*B+C)
      | P-((D-A)*B+C+CARRYIN)
      | P-((D-A)*B+CARRYIN)
      | P-(C+(D-A)*B+CARRYIN)
      | P-(P+(D-A)*B+CARRYIN)
      | P>>17+(D-A)*B+C
      | P>>17+(D-A)*B+C+CARRYIN
      | P>>17+(D-A)*B+CARRYIN
      | P>>17+C+(D-A)*B+CARRYIN
      | P>>17+P+(D-A)*B+CARRYIN
      | P>>17-((D-A)*B+C)
      | P>>17-((D-A)*B+C+CARRYIN)
      | P>>17-((D-A)*B+CARRYIN)
      | P>>17-(C+(D-A)*B+CARRYIN)
      | P>>17-(P+(D-A)*B+CARRYIN)
      | PCIN+(D-A)*B+C
      | PCIN+(D-A)*B+C+CARRYIN
      | PCIN+(D-A)*B+CARRYIN
      | PCIN+C+(D-A)*B+CARRYIN
      | PCIN+P+(D-A)*B+CARRYIN
      | PCIN-((D-A)*B+C)
      | PCIN-((D-A)*B+C+CARRYIN)
      | PCIN-((D-A)*B+CARRYIN)
      | PCIN-(C+(D-A)*B+CARRYIN)
      | PCIN-(P+(D-A)*B+CARRYIN)
      | PCIN>>17+(D-A)*B+C
      | PCIN>>17+(D-A)*B+C+CARRYIN
      | PCIN>>17+(D-A)*B+CARRYIN
      | PCIN>>17+C+(D-A)*B+CARRYIN
      | PCIN>>17+P+(D-A)*B+CARRYIN
      | PCIN>>17-((D-A)*B+C)
      | PCIN>>17-((D-A)*B+C+CARRYIN)
      | PCIN>>17-((D-A)*B+CARRYIN)
      | PCIN>>17-(C+(D-A)*B+CARRYIN)
      | PCIN>>17-(P+(D-A)*B+CARRYIN)
      | RNDMACC((D-A)*B+C+P)
      | RNDSIMPLE((D-A)*B+C)
      | RNDSIMPLE((D-A)*B+C+CARRYIN)
      | RNDSIMPLE((D-A)*B+CARRYIN)
      | RNDSIMPLE(C+(D-A)*B+CARRYIN)
      | RNDSIMPLE(P+(D-A)*B+CARRYIN)
      | RNDSIMPLE(P>>17+(D-A)*B+CARRYIN)
      | RNDSIMPLE(PCIN+(D-A)*B+CARRYIN)
      | RNDSIMPLE(PCIN>>17+(D-A)*B+CARRYIN)
      settings: infoedit=<html>Valid operands: CONCAT, P, C, PCIN, P>>17, PCIN>>17, CARRYIN, CARRYCASCIN, ACIN, A, BCIN,B<br><br>Valid operators: +, -, *, ()<br><br>Valid functions: RNDSIMPLE, RNDSYM<br><br>Instructions are case insensitive and tolerate spaces.</html>
  Convert : xbsIndex_r4/Convert  gui_display_data_type=Fixed-point  arith_type=Unsigned  n_bits=24  bin_pt=0  float_type=Single  exp_bits=8  fraction_bits=24  quantization=Truncate  overflow=Wrap  en=off  latency=0  pipeline=off  dbl_ovrd=off  block_type=convert
  Convert1 : xbsIndex_r4/Convert  gui_display_data_type=Fixed-point  arith_type="Signed  (2's comp)"  n_bits=25  bin_pt=0  float_type=Single  exp_bits=8  fraction_bits=24  quantization=Truncate  overflow=Wrap  en=off  latency=0  pipeline=off  dbl_ovrd=off  block_type=convert
  Convert2 : xbsIndex_r4/Convert  gui_display_data_type=Fixed-point  arith_type="Signed  (2's comp)"  n_bits=18  bin_pt=15  float_type=Single  exp_bits=8  fraction_bits=24  quantization=Truncate  overflow=Wrap  en=off  latency=0  pipeline=off  dbl_ovrd=off  block_type=convert
  Convert3 : xbsIndex_r4/Convert  gui_display_data_type=Fixed-point  arith_type="Signed  (2's comp)"  n_bits=25  bin_pt=0  float_type=Single  exp_bits=8  fraction_bits=24  quantization=Truncate  overflow=Wrap  en=off  latency=0  pipeline=off  dbl_ovrd=off  block_type=convert
  Delay : xbsIndex_r4/Delay  rst=off  infoeditControl=Selection of Reset will increase slice count due to use of real FFs and instead of SRLs  en=off  latency=4  reg_retiming=off  dbl_ovrd=off  block_type=delay
  Delay1 : xbsIndex_r4/Delay  rst=off  infoeditControl=Selection of Reset will increase slice count due to use of real FFs and instead of SRLs  en=off  latency=4  reg_retiming=off  dbl_ovrd=off  block_type=delay
  Register : xbsIndex_r4/Register  init=0  rst=off  en=off  dbl_ovrd=off  block_type=register
  Out1 : Outport
  ch_o : Outport  Port=2
  wires:
  Register/1 -> Convert3/1
  In1/1 -> Register/1
  Delay/1 -> Convert1/1, (D-A)*B + C/4
  (D-A)*B + C/1 -> Convert/1, Delay/1
  Convert1/1 -> (D-A)*B + C/2
  Convert/1 -> Out1/1
  Convert2/1 -> (D-A)*B + C/3
  Convert3/1 -> (D-A)*B + C/1
  ch/1 -> Delay1/1
  Delay1/1 -> ch_o/1
  alpha/1 -> Convert2/1

== system CryoDetHcd/DspCore/DSP/channel_processor/channel_processor_x4/dF_debug/alpha_filter3 ==
  In1 : Inport
  alpha : Inport  Port=2
  ch : Inport  Port=3
  (D-A)*B + C : xbsIndex_r4/DSP48 Macro 3.0   dsptype=Target XtremeDSP Slice: DSP48E2  instruction_list=(D-A)*B+C  AvailableInstructions=|  show_filtered=on  pipeline_options=Expert  dspimage=?  tier_1=off  tier_2=off  tier_3=off  tier_4=off  tier_5=off  tier_6=off  dreg_1=off  dreg_2=off  dreg_3=on  areg_1=off  areg_2=off  areg_3=on  areg_4=on  breg_1=off  breg_2=off  breg_3=on  breg_4=on  mreg_5=on  concatreg_3=off  concatreg_4=off  concatreg_5=off  creg_1=off  creg_2=off  creg_3=on  creg_4=on  creg_5=on  preg_6=on  cinreg_1=off  cinreg_2=off  cinreg_3=off  cinreg_4=off  cinreg_5=off  opreg_1=off  opreg_2=off  opreg_3=off  opreg_4=off  opreg_5=off  output_properties=Full_Precision  p_width=48  p_binarywidth=0  has_acout=off  has_bcout=off  has_pcout=off  has_carryout=off  has_carrycascout=off  has_ce=off  has_d_ce=off  has_a_ce=off  has_b_ce=off  has_concat_ce=off  has_c_ce=off  has_m_ce=off  has_p_ce=off  has_sel_ce=off  has_sclr=off  has_d_sclr=off  has_a_sclr=off  has_b_sclr=off  has_concat_sclr=off  has_c_sclr=off  has_m_sclr=off  has_p_sclr=off  has_sel_sclr=off  use_dsp48=on  simulation_type=fast_sim  simulation_model=sysgen:xbip_dsp48_macro_v3_0  gui_behaviour=Sysgen  instruction1='#'  ip_name=DSP48 Macro  ip_version=3.0  dsptool_ready=true  ipcore_usecache=true  ipcore_useipmodelcache=true  wrapper_available=true  port_translation_map={ 'ce' => 'en', 'sclr' => 'rst'}  ipcore_latency_function='has_combinational'  structural_sim=false  ipcore_verbose=false  ipcore_port_config={ 'carryin' => { 'arith' => 'ufix', 'binpt' => 0.00000000000, 'width' => 1.00000000000}, 'carrycascin' => { 'arith' => 'ufix', 'binpt' => 0.00000000000, 'width' => 1.00000000000}, 'carrycascout' => { 'arith' => 'ufix', 'binpt' => 0.00000000000, 'width' => 1.00000000000}, 'carryout' => { 'arith' => 'ufix', 'binpt' => 0.00000000000, 'width' => 1.00000000000}}  ipcore_xco_need_fpga_part=true  block_type=xbip_dsp48_macro_v3_0
      | (D-A)*B+C
      | (D-A)*B+C+C
      | (D-A)*B+C+C+CARRYIN
      | (D-A)*B+C+CARRYIN
      | (D-A)*B+C+P
      | (D-A)*B+C+P+CARRYIN
      | (D-A)*B+C+P>>17
      | (D-A)*B+C+P>>17+CARRYIN
      | (D-A)*B+C+PCIN
      | (D-A)*B+C+PCIN+CARRYIN
      | (D-A)*B+C+PCIN>>17
      | (D-A)*B+C+PCIN>>17+CARRYIN
      | (D-A)*B+C-C
      | (D-A)*B+C-P
      | (D-A)*B+C-P>>17
      | (D-A)*B+C-PCIN
      | (D-A)*B+C-PCIN>>17
      | (D-A)*B+CARRYIN
      | -((D-A)*B+C)
      | -((D-A)*B+C+CARRYIN)
      | -((D-A)*B+CARRYIN)
      | -(C+(D-A)*B+CARRYIN)
      | -(P+(D-A)*B+CARRYIN)
      | -C+(D-A)*B+C
      | -P+(D-A)*B+C
      | -P>>17+(D-A)*B+C
      | -PCIN+(D-A)*B+C
      | -PCIN>>17+(D-A)*B+C
      | C+(D-A)*B+C
      | C+(D-A)*B+C+CARRYIN
      | C+(D-A)*B+CARRYIN
      | C+C+(D-A)*B+CARRYIN
      | C+P+(D-A)*B+CARRYIN
      | C+P>>17+(D-A)*B+CARRYIN
      | C+PCIN+(D-A)*B+CARRYIN
      | C+PCIN>>17+(D-A)*B+CARRYIN
      | C-((D-A)*B+C)
      | C-((D-A)*B+C+CARRYIN)
      | C-((D-A)*B+CARRYIN)
      | C-(C+(D-A)*B+CARRYIN)
      | C-(P+(D-A)*B+CARRYIN)
      | P+(D-A)*B+C
      | P+(D-A)*B+C+CARRYIN
      | P+(D-A)*B+CARRYIN
      | P+C+(D-A)*B+CARRYIN
      | P+P+(D-A)*B+CARRYIN
      | P+P>>17+(D-A)*B+CARRYIN
      | P+PCIN+(D-A)*B+CARRYIN
      | P+PCIN>>17+(D-A)*B+CARRYIN
      | P-((D-A)*B+C)
      | P-((D-A)*B+C+CARRYIN)
      | P-((D-A)*B+CARRYIN)
      | P-(C+(D-A)*B+CARRYIN)
      | P-(P+(D-A)*B+CARRYIN)
      | P>>17+(D-A)*B+C
      | P>>17+(D-A)*B+C+CARRYIN
      | P>>17+(D-A)*B+CARRYIN
      | P>>17+C+(D-A)*B+CARRYIN
      | P>>17+P+(D-A)*B+CARRYIN
      | P>>17-((D-A)*B+C)
      | P>>17-((D-A)*B+C+CARRYIN)
      | P>>17-((D-A)*B+CARRYIN)
      | P>>17-(C+(D-A)*B+CARRYIN)
      | P>>17-(P+(D-A)*B+CARRYIN)
      | PCIN+(D-A)*B+C
      | PCIN+(D-A)*B+C+CARRYIN
      | PCIN+(D-A)*B+CARRYIN
      | PCIN+C+(D-A)*B+CARRYIN
      | PCIN+P+(D-A)*B+CARRYIN
      | PCIN-((D-A)*B+C)
      | PCIN-((D-A)*B+C+CARRYIN)
      | PCIN-((D-A)*B+CARRYIN)
      | PCIN-(C+(D-A)*B+CARRYIN)
      | PCIN-(P+(D-A)*B+CARRYIN)
      | PCIN>>17+(D-A)*B+C
      | PCIN>>17+(D-A)*B+C+CARRYIN
      | PCIN>>17+(D-A)*B+CARRYIN
      | PCIN>>17+C+(D-A)*B+CARRYIN
      | PCIN>>17+P+(D-A)*B+CARRYIN
      | PCIN>>17-((D-A)*B+C)
      | PCIN>>17-((D-A)*B+C+CARRYIN)
      | PCIN>>17-((D-A)*B+CARRYIN)
      | PCIN>>17-(C+(D-A)*B+CARRYIN)
      | PCIN>>17-(P+(D-A)*B+CARRYIN)
      | RNDMACC((D-A)*B+C+P)
      | RNDSIMPLE((D-A)*B+C)
      | RNDSIMPLE((D-A)*B+C+CARRYIN)
      | RNDSIMPLE((D-A)*B+CARRYIN)
      | RNDSIMPLE(C+(D-A)*B+CARRYIN)
      | RNDSIMPLE(P+(D-A)*B+CARRYIN)
      | RNDSIMPLE(P>>17+(D-A)*B+CARRYIN)
      | RNDSIMPLE(PCIN+(D-A)*B+CARRYIN)
      | RNDSIMPLE(PCIN>>17+(D-A)*B+CARRYIN)
      settings: infoedit=<html>Valid operands: CONCAT, P, C, PCIN, P>>17, PCIN>>17, CARRYIN, CARRYCASCIN, ACIN, A, BCIN,B<br><br>Valid operators: +, -, *, ()<br><br>Valid functions: RNDSIMPLE, RNDSYM<br><br>Instructions are case insensitive and tolerate spaces.</html>
  Convert : xbsIndex_r4/Convert  gui_display_data_type=Fixed-point  arith_type=Unsigned  n_bits=24  bin_pt=0  float_type=Single  exp_bits=8  fraction_bits=24  quantization=Truncate  overflow=Wrap  en=off  latency=0  pipeline=off  dbl_ovrd=off  block_type=convert
  Convert1 : xbsIndex_r4/Convert  gui_display_data_type=Fixed-point  arith_type="Signed  (2's comp)"  n_bits=25  bin_pt=0  float_type=Single  exp_bits=8  fraction_bits=24  quantization=Truncate  overflow=Wrap  en=off  latency=0  pipeline=off  dbl_ovrd=off  block_type=convert
  Convert2 : xbsIndex_r4/Convert  gui_display_data_type=Fixed-point  arith_type="Signed  (2's comp)"  n_bits=18  bin_pt=15  float_type=Single  exp_bits=8  fraction_bits=24  quantization=Truncate  overflow=Wrap  en=off  latency=0  pipeline=off  dbl_ovrd=off  block_type=convert
  Convert3 : xbsIndex_r4/Convert  gui_display_data_type=Fixed-point  arith_type="Signed  (2's comp)"  n_bits=25  bin_pt=0  float_type=Single  exp_bits=8  fraction_bits=24  quantization=Truncate  overflow=Wrap  en=off  latency=0  pipeline=off  dbl_ovrd=off  block_type=convert
  Delay : xbsIndex_r4/Delay  rst=off  infoeditControl=Selection of Reset will increase slice count due to use of real FFs and instead of SRLs  en=off  latency=4  reg_retiming=off  dbl_ovrd=off  block_type=delay
  Delay1 : xbsIndex_r4/Delay  rst=off  infoeditControl=Selection of Reset will increase slice count due to use of real FFs and instead of SRLs  en=off  latency=4  reg_retiming=off  dbl_ovrd=off  block_type=delay
  Register : xbsIndex_r4/Register  init=0  rst=off  en=off  dbl_ovrd=off  block_type=register
  Out1 : Outport
  ch_o : Outport  Port=2
  wires:
  alpha/1 -> Convert2/1
  Delay1/1 -> ch_o/1
  ch/1 -> Delay1/1
  Convert3/1 -> (D-A)*B + C/1
  Convert2/1 -> (D-A)*B + C/3
  Convert/1 -> Out1/1
  Convert1/1 -> (D-A)*B + C/2
  (D-A)*B + C/1 -> Delay/1, Convert/1
  Delay/1 -> (D-A)*B + C/4, Convert1/1
  In1/1 -> Register/1
  Register/1 -> Convert3/1
